simulink model "ModelDosingUnit"  (R2020b)
settings: Solver=FixedStepAuto  StartTime=0.0  StopTime=Inf  FixedStep=0.010  RelTol=1e-3
settings Model: Creator=kaebi  LastModifiedBy=kaebi
settings OptimizationCC: DefaultParameterBehavior=Inlined  LocalBlockOutputs=off
settings RTWCC: Description=TwinCAT GRT Target  SystemTargetFile=TwinCatGrt.tlc  GenCodeOnly=on  TemplateMakefile=tcgrt_msbuild.tmf  TargetLang=C++
settings STFCustomTargetCC: TargetLangStandard=C++03 (ISO)  ConcurrentExecutionCompliant=off  CombineOutputUpdateFcns=on  CodeInterfacePackaging=Reusable function  GRTInterface=off  GenerateAllocFcn=on  SystemTargetFile=TwinCatGrt.tlc
settings GRTTargetCC: TargetLangStandard=C++03 (ISO)  ParMdlRefBuildCompliant=off  CompOptLevelCompliant=off  ConcurrentExecutionCompliant=off  MatFileLogging=off  CodeInterfacePackaging=Reusable function  GenerateAllocFcn=on  UseToolchainInfoCompliant=off  ExtModeMexFile=TcExtModeClient

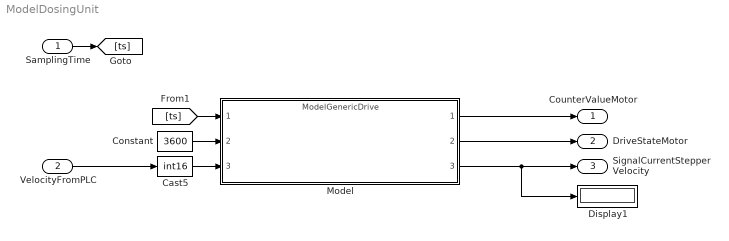
== system ModelDosingUnit ==
  SamplingTime : Inport
  VelocityFromPLC : Inport  Port=2  OutDataTypeStr=uint32
  Cast5 : DataTypeConversion  OutDataTypeStr=int16
  Constant : Constant  Value=3600
  Display1 : Display
      settings: Format=decimal (Stored Integer)
  Model : ModelReference  ModelNameDialog=ModelGenericDrive.slx  SimulationMode=Normal  ModelReferenceVersion=1.12
  CounterValueMotor : Outport
  DriveStateMotor : Outport  Port=2
  SignalCurrentStepperVelocity : Outport  Port=3
  wires:
  Model/3 -> Display1/1, SignalCurrentStepperVelocity/1
  Model/2 -> DriveStateMotor/1
  VelocityFromPLC/1 -> Cast5/1
  Model/1 -> CounterValueMotor/1
  SamplingTime/1 -> [ts]
  Constant/1 -> Model/2
  [ts] -> Model/1
  Cast5/1 -> Model/3
